simulink model "gm_sampleModel1948_1_sub"  (R2023a)
settings: Solver=VariableStepAuto  StartTime=0.0  StopTime=10.0  RelTol=1e-3
libraries: simulink x3
settings Model: Creator=user1  LastModifiedBy=user1
settings OptimizationCC: BlockReduction=off  ConditionallyExecuteInputs=off
settings DebuggingCC: InheritedTsInSrcMsg=none

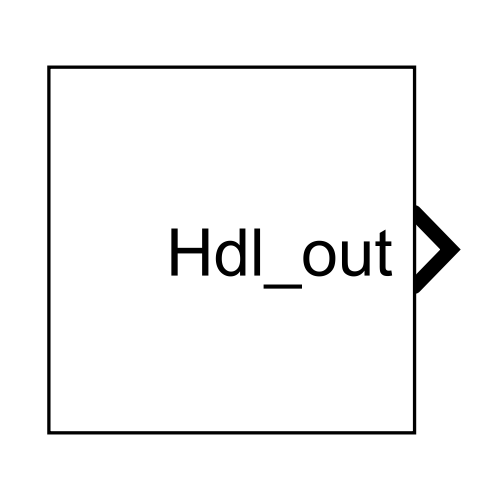
[thumbnail: Simulink's stored preview of the top-level diagram]
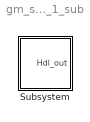
== system gm_sampleModel1948_1_sub ==
  Subsystem : Subsystem

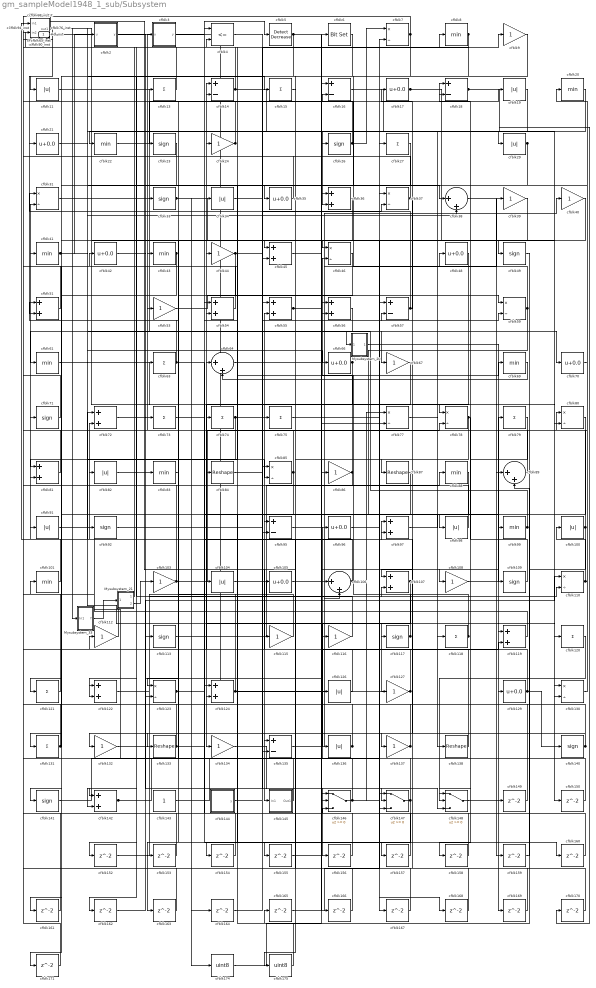
== system gm_sampleModel1948_1_sub/Subsystem ==
  Mysubsystem_20 : Subsystem
  Mysubsystem_21 : Subsystem
  Mysubsystem_33 : Subsystem
  cfblk{11,19,29,34,82,91,98,100,104,126,136} (11 alike) : Abs  OutDataTypeStr=uint8  SaturateOnIntegerOverflow=off
  cfblk{8,20,22,41,43,61,69,83,88,99,101} (11 alike) : MinMax  OutDataTypeStr=uint8
  cfblk102_inst : Subsystem
  cfblk{9,24,39..40,44,53,67,86,103,108,112,115..116,127,132,134,137} (17 alike) : Gain  OutDataTypeStr=uint8
  cfblk{17,21,35,42,48,66,70,96,105,129} (10 alike) : Bias  Bias=0.0  SaturateOnIntegerOverflow=off
  cfblk{38,64,89,106} (4 alike) : Sum  Inputs=|++  OutDataTypeStr=uint8
  cfblk{36,45,51,54..56,72,81,97,107,119,122,124,142} (14 alike) : Sum  OutDataTypeStr=uint8
  cfblk{23,26,33,49,71,92,109,113,117,140..141} (11 alike) : Signum
  cfblk10_inst : Subsystem
  cfblk{7,31,37,46,59,77..78,80,85,110,123,130} (12 alike) : Product  Inputs=*/  OutDataTypeStr=uint8  RndMeth=Zero  SaturateOnIntegerOverflow=on
  cfblk111_inst : Subsystem
  cfblk{13,15,27,63,73..75,79,118,120..121,131} (12 alike) : Sum  Inputs=+  OutDataTypeStr=uint8
  cfblk125_inst : Subsystem
  cfblk128_inst : Subsystem
  cfblk12_inst : Subsystem
  cfblk{84,87,133,138} (4 alike) : Reshape
  cfblk{14,16,18,57,95,135} (6 alike) : Sum  Inputs=+-  OutDataTypeStr=uint8
  cfblk139_inst : Subsystem
  cfblk143 : Constant  OutDataTypeStr=uint8  SampleTime=-1
  cfblk144 : Subsystem  mask(Counter Free-Running){NumBits=double(16), tsamp=double(-1)}
      mask prompts: NumBits "Simulink:masks:NumberOfBits_MP"; tsamp "Simulink:masks:SampleTime_MP"
      mask help: Simulink:masks:CounterFreeRunning_MD
  cfblk145 : Subsystem
  cfblk146 : Switch  OutDataTypeStr=uint8  SaturateOnIntegerOverflow=off  InputSameDT=off
  cfblk147 : Switch  OutDataTypeStr=uint8  SaturateOnIntegerOverflow=off  InputSameDT=off
  cfblk148 : Switch  OutDataTypeStr=uint8  SaturateOnIntegerOverflow=off  InputSameDT=off
  cfblk{149..150,152..171} (22 alike) : Delay  SampleTime=1
  cfblk174 : DataTypeConversion  OutDataTypeStr=uint8  SaturateOnIntegerOverflow=off  RndMeth=Floor
  cfblk175 : DataTypeConversion  OutDataTypeStr=uint8  SaturateOnIntegerOverflow=off  RndMeth=Floor
  cfblk2 : Subsystem  mask(Compare To Constant){relop=<=, const=double(3), OutDataTypeStr=uint8, ZeroCross=on}
      mask prompts: relop "Simulink:masks:Operator_MP"; const "Simulink:masks:ConstantValue_MP"; OutDataTypeStr "Simulink:masks:OutputDataType_MP"; ZeroCross "Simulink:masks:EnableZerocrossingDetection_MP"
      mask help: Simulink:masks:CompareToConstant_MD
      mask init:
      | OutDataTypeStr = 'uint8';
      | ZeroCross = 'on';
      | blkName = 'sampleModel1948_1_sub/Subsystem/cfblk2';
      | const = double(3);
      | const_str = '3.0';
      | const_val = double(3);
      | relop = '<=';
      | setValue = 'fixdt(0, 8)';
      | str = '<= 3';
      mask TypeOptions relop: == | ~= | < | <= | >= | >
      mask TypeOptions OutDataTypeStr: Simulink:masks:uint8 | Simulink:masks:boolean
      mask Callback ZeroCross: sl('zeroCrossEnable', gcbh);
      mask Display: disp(str)
  cfblk28_inst : Subsystem
  cfblk3 : Subsystem  mask(Compare To Constant){relop=<=, const=double(3), OutDataTypeStr=uint8, ZeroCross=on}
      mask prompts: relop "Simulink:masks:Operator_MP"; const "Simulink:masks:ConstantValue_MP"; OutDataTypeStr "Simulink:masks:OutputDataType_MP"; ZeroCross "Simulink:masks:EnableZerocrossingDetection_MP"
      mask help: Simulink:masks:CompareToConstant_MD
      mask init:
      | OutDataTypeStr = 'uint8';
      | ZeroCross = 'on';
      | blkName = 'sampleModel1948_1_sub/Subsystem/cfblk3';
      | const = double(3);
      | const_str = '3.0';
      | const_val = double(3);
      | relop = '<=';
      | setValue = 'fixdt(0, 8)';
      | str = '<= 3';
      mask TypeOptions relop: == | ~= | < | <= | >= | >
      mask TypeOptions OutDataTypeStr: Simulink:masks:uint8 | Simulink:masks:boolean
      mask Callback ZeroCross: sl('zeroCrossEnable', gcbh);
      mask Display: disp(str)
  cfblk30_inst : Subsystem
  cfblk32_inst : Subsystem
  cfblk4 : RelationalOperator  Operator=<=  OutDataTypeStr=boolean  InputSameDT=off
  cfblk47_inst : Subsystem
  cfblk5 : simulink/Logic and Bit Operations/Detect Decrease  vinit=0.0  OutDataTypeStr=uint8
      settings: LibrarySourceBlock=|
      | hdlsllib/Logic and Bit
      | Operations/Detect
      | Decrease
  cfblk58_inst : Subsystem
  cfblk6 : simulink/Logic and Bit Operations/Bit Set  iBit=0
      settings: LibrarySourceBlock=|
      | hdlsllib/Logic and Bit
      | Operations/Bit Set
  cfblk60_inst : Subsystem
  cfblk62_inst : Subsystem
  cfblk65_inst : Subsystem
  cfblk68_inst : Subsystem
  cfblk76_inst : Subsystem
  cfblk90_inst : Subsystem
  cfblk94_inst : Subsystem
  Hdl_out : Outport  OutDataTypeStr=uint8  SampleTime=1
  wires:
  Mysubsystem_20/1(Out1) -> cfblk169/1
  Mysubsystem_21/1(Out1) -> cfblk60_inst/2(in2)
  Mysubsystem_21/2(Out2) -> cfblk103/1
  Mysubsystem_33/1(Y) -> Mysubsystem_21/1(In1)
  cfblk10_inst/1(out1) -> cfblk11/1
  cfblk100/1 -> cfblk165/1, cfblk3/1(u)
  cfblk101/1 -> cfblk62_inst/1(in1)
  cfblk102_inst/1(out1) -> cfblk145/1(In1)
  cfblk103/1 -> cfblk94_inst/1(in1), cfblk78/2
  cfblk104/1 -> cfblk107/2
  cfblk105/1 -> cfblk40/1
  cfblk106/1 -> cfblk72/2, cfblk31/2
  cfblk107/1 -> cfblk155/1, cfblk134/1
  cfblk108/1 -> cfblk79/1
  cfblk109/1 -> cfblk48/1
  cfblk11/1 -> cfblk70/1
  cfblk110/1 -> cfblk35/1, cfblk100/1
  cfblk111_inst/1(out1) -> cfblk139_inst/1(in1), cfblk124/2
  cfblk112/1 -> cfblk47_inst/1(in1)
  cfblk113/1 -> cfblk88/1
  cfblk115/1 -> cfblk53/1
  cfblk116/1 -> cfblk58_inst/1(in1)
  cfblk117/1 -> cfblk42/1, cfblk31/1
  cfblk118/1 -> cfblk111_inst/1(in1), cfblk46/2
  cfblk119/1 -> cfblk101/1
  cfblk12_inst/1(out1) -> cfblk73/1
  cfblk120/1 -> cfblk148/2
  cfblk121/1 -> cfblk12_inst/1(in1)
  cfblk122/1 -> cfblk110/2
  cfblk123/1 -> cfblk174/1, cfblk157/1
  cfblk124/1 -> cfblk14/1, cfblk106/2
  cfblk125_inst/1(out1) -> cfblk49/1
  cfblk126/1 -> cfblk128_inst/1(in1)
  cfblk127/1 -> cfblk55/2, cfblk30_inst/1(in1), cfblk44/1, Hdl_out/1
  cfblk128_inst/1(out1) -> Mysubsystem_33/1(In1)
  cfblk129/1 -> cfblk54/2, cfblk140/1
  cfblk13/1 -> cfblk65_inst/1(in1)
  cfblk130/1 -> cfblk80/1
  cfblk131/1 -> cfblk128_inst/2(in2), cfblk41/1
  cfblk132/1 -> cfblk4/1
  cfblk133/1 -> cfblk97/1, cfblk71/1
  cfblk134/1 -> cfblk156/1
  cfblk135/1 -> cfblk39/1
  cfblk136/1 -> cfblk30_inst/2(in2), cfblk135/1
  cfblk137/1 -> cfblk94_inst/2(in2), cfblk91/1, cfblk24/1
  cfblk138/1 -> cfblk82/1
  cfblk139_inst/1(out1) -> cfblk86/1
  cfblk14/1 -> cfblk76_inst/2(in2), cfblk29/1
  cfblk140/1 -> cfblk132/1, cfblk43/1
  cfblk141/1 -> cfblk45/2
  cfblk142/1 -> cfblk96/1, cfblk57/1
  cfblk143/1 -> cfblk56/1
  cfblk144/1(y) -> cfblk59/2
  cfblk145/1(Out1) -> cfblk72/1
  cfblk146/1 -> cfblk12_inst/2(in2), cfblk77/1, cfblk7/2, cfblk27/1
  cfblk147/1 -> cfblk106/1, cfblk163/1, cfblk13/1
  cfblk148/1 -> cfblk149/1
  cfblk149/1 -> cfblk139_inst/2(in2)
  cfblk15/1 -> cfblk45/1
  cfblk150/1 -> cfblk111_inst/2(in2)
  cfblk152/1 -> cfblk64/1
  cfblk153/1 -> cfblk62_inst/2(in2)
  cfblk154/1 -> cfblk124/1
  cfblk155/1 -> cfblk119/2
  cfblk156/1 -> cfblk146/3
  cfblk157/1 -> cfblk14/2
  cfblk158/1 -> cfblk32_inst/2(in2)
  cfblk159/1 -> cfblk89/2
  cfblk16/1 -> cfblk120/1
  cfblk160/1 -> cfblk76_inst/1(in1)
  cfblk161/1 -> cfblk60_inst/1(in1)
  cfblk162/1 -> cfblk110/1
  cfblk163/1 -> cfblk90_inst/2(in2)
  cfblk164/1 -> cfblk57/2
  cfblk165/1 -> cfblk37/1
  cfblk166/1 -> cfblk125_inst/2(in2)
  cfblk167/1 -> cfblk95/1
  cfblk168/1 -> cfblk146/1
  cfblk169/1 -> cfblk4/2
  cfblk17/1 -> cfblk89/1, cfblk130/2
  cfblk170/1 -> cfblk97/2
  cfblk171/1 -> cfblk58_inst/2(in2)
  cfblk174/1 -> cfblk6/1
  cfblk175/1 -> cfblk104/1
  cfblk18/1 -> cfblk170/1, cfblk130/1
  cfblk19/1 -> cfblk122/2
  cfblk2/1(y) -> cfblk147/2
  cfblk20/1 -> cfblk22/1
  cfblk21/1 -> cfblk66/1
  cfblk22/1 -> cfblk19/1
  cfblk23/1 -> cfblk161/1
  cfblk24/1 -> cfblk68_inst/2(in2), cfblk10_inst/2(in2)
  cfblk26/1 -> cfblk125_inst/1(in1), cfblk7/1
  cfblk27/1 -> cfblk84/1
  cfblk28_inst/1(out1) -> cfblk92/1, cfblk36/2, cfblk123/2
  cfblk29/1 -> cfblk135/2, cfblk152/1
  cfblk3/1(y) -> cfblk5/1
  cfblk30_inst/1(out1) -> cfblk75/1
  cfblk31/1 -> cfblk56/2
  cfblk32_inst/1(out1) -> cfblk118/1
  cfblk33/1 -> cfblk147/1, cfblk164/1
  cfblk34/1 -> cfblk78/1
  cfblk35/1 -> cfblk23/1
  cfblk36/1 -> cfblk81/1
  cfblk37/1 -> cfblk90_inst/1(in1), cfblk87/1
  cfblk38/1 -> cfblk80/2
  cfblk39/1 -> cfblk153/1
  cfblk4/1 -> cfblk119/1
  cfblk40/1 -> cfblk46/1
  cfblk41/1 -> cfblk166/1, cfblk2/1(u)
  cfblk42/1 -> cfblk113/1
  cfblk43/1 -> cfblk142/1, cfblk171/1
  cfblk44/1 -> cfblk133/1, cfblk8/1
  cfblk45/1 -> cfblk108/1
  cfblk46/1 -> cfblk123/1
  cfblk47_inst/1(out1) -> cfblk102_inst/2(in2), cfblk150/1
  cfblk48/1 -> cfblk137/1
  cfblk49/1 -> cfblk129/1
  cfblk5/1 -> cfblk77/2, cfblk162/1
  cfblk51/1 -> cfblk10_inst/1(in1)
  cfblk53/1 -> cfblk59/1
  cfblk54/1 -> cfblk68_inst/1(in1)
  cfblk55/1 -> cfblk109/1, cfblk9/1
  cfblk56/1 -> cfblk61/1
  cfblk57/1 -> cfblk34/1, cfblk17/1
  cfblk58_inst/1(out1) -> cfblk26/1
  cfblk59/1 -> cfblk95/2, cfblk16/2
  cfblk6/1 -> cfblk175/1
  cfblk60_inst/1(out1) -> cfblk51/2, cfblk147/3, cfblk136/1, cfblk115/1
  cfblk61/1 -> cfblk159/1
  cfblk62_inst/1(out1) -> cfblk38/2, cfblk127/1
  cfblk63/1 -> cfblk98/1, cfblk51/1
  cfblk64/1 -> cfblk116/1
  cfblk65_inst/1(out1) -> cfblk15/1
  cfblk66/1 -> cfblk54/1, cfblk74/1
  cfblk67/1 -> cfblk146/2
  cfblk68_inst/1(out1) -> cfblk85/2, cfblk167/1
  cfblk69/1 -> cfblk64/2
  cfblk7/1 -> cfblk36/1, cfblk28_inst/1(in1), cfblk142/2
  cfblk70/1 -> cfblk20/1
  cfblk71/1 -> cfblk32_inst/1(in1)
  cfblk72/1 -> cfblk126/1
  cfblk73/1 -> cfblk160/1
  cfblk74/1 -> cfblk37/2, cfblk121/1
  cfblk75/1 -> cfblk18/1
  cfblk76_inst/1(out1) -> cfblk38/1, cfblk67/1
  cfblk77/1 -> cfblk138/1
  cfblk78/1 -> cfblk105/1, cfblk158/1
  cfblk79/1 -> cfblk148/1
  cfblk8/1 -> cfblk28_inst/2(in2), cfblk141/1
  cfblk80/1 -> cfblk122/1
  cfblk81/1 -> cfblk47_inst/2(in2)
  cfblk82/1 -> cfblk83/1
  cfblk83/1 -> cfblk33/1
  cfblk84/1 -> cfblk148/3
  cfblk85/1 -> cfblk102_inst/1(in1), cfblk154/1
  cfblk86/1 -> cfblk81/2, cfblk65_inst/2(in2)
  cfblk87/1 -> cfblk131/1
  cfblk88/1 -> cfblk107/1
  cfblk89/1 -> cfblk55/1
  cfblk9/1 -> cfblk112/1
  cfblk90_inst/1(out1) -> cfblk63/1
  cfblk91/1 -> cfblk117/1
  cfblk92/1 -> cfblk85/1
  cfblk94_inst/1(out1) -> cfblk21/1
  cfblk95/1 -> cfblk69/1
  cfblk96/1 -> cfblk168/1
  cfblk97/1 -> cfblk99/1
  cfblk98/1 -> cfblk16/1
  cfblk99/1 -> cfblk18/2, Mysubsystem_20/1(In1)

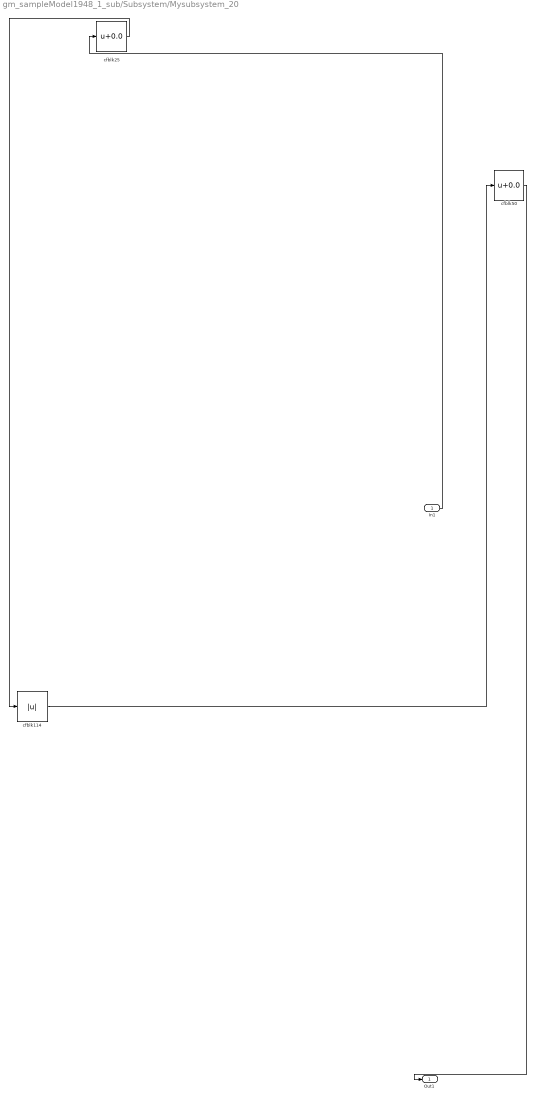
== system gm_sampleModel1948_1_sub/Subsystem/Mysubsystem_20 ==
  In1 : Inport  OutDataTypeStr=uint8  PortDimensions=1  SampleTime=1
  cfblk114 : Abs  SaturateOnIntegerOverflow=off
  cfblk25 : Bias  Bias=0.0  SaturateOnIntegerOverflow=off
  cfblk50 : Bias  Bias=0.0  SaturateOnIntegerOverflow=off
  Out1 : Outport  SampleTime=1
  wires:
  In1/1 -> cfblk25/1
  cfblk114/1 -> cfblk50/1
  cfblk25/1 -> cfblk114/1
  cfblk50/1 -> Out1/1

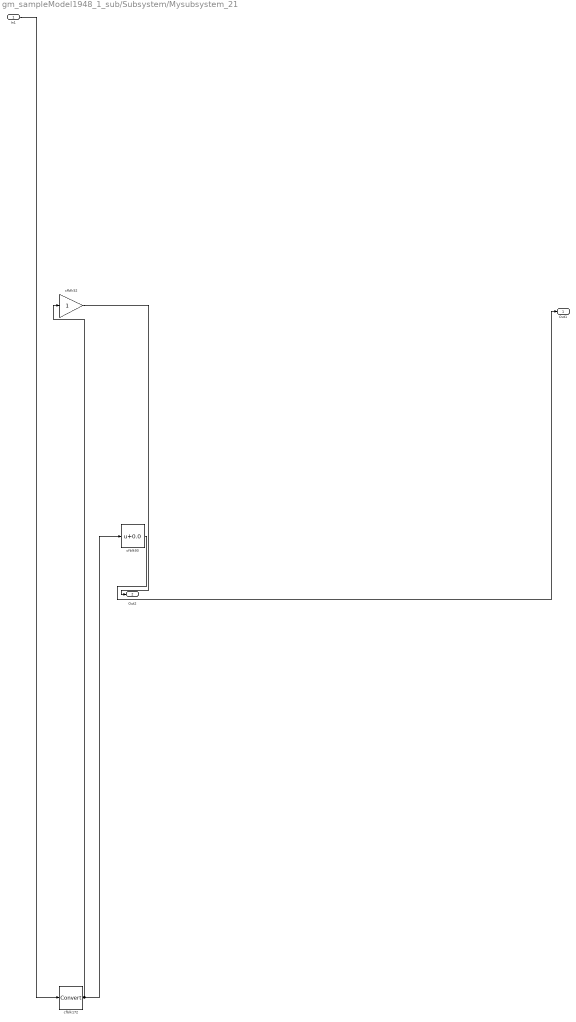
== system gm_sampleModel1948_1_sub/Subsystem/Mysubsystem_21 ==
  In1 : Inport  OutDataTypeStr=boolean  PortDimensions=1  SampleTime=1
  cfblk172 : DataTypeConversion  SaturateOnIntegerOverflow=off  RndMeth=Floor
  cfblk52 : Gain
  cfblk93 : Bias  Bias=0.0  SaturateOnIntegerOverflow=off
  Out1 : Outport  SampleTime=1
  Out2 : Outport  Port=2  SampleTime=1
  wires:
  In1/1 -> cfblk172/1
  cfblk172/1 -> cfblk93/1, cfblk52/1
  cfblk52/1 -> Out2/1
  cfblk93/1 -> Out1/1

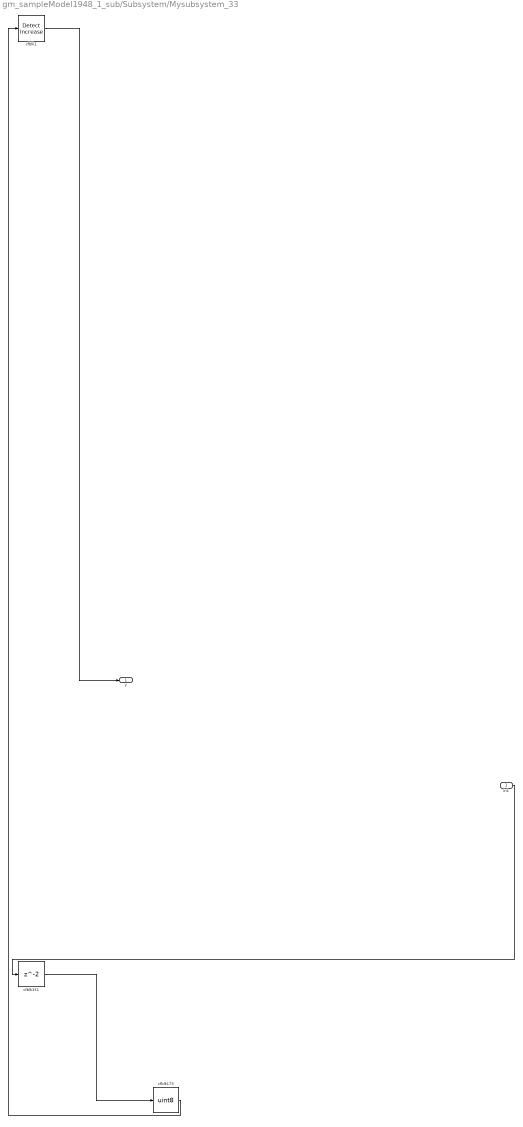
== system gm_sampleModel1948_1_sub/Subsystem/Mysubsystem_33 ==
  In1 : Inport  OutDataTypeStr=uint8  PortDimensions=1  SampleTime=1
  cfblk1 : simulink/Logic and Bit Operations/Detect Increase  vinit=0.0  OutDataTypeStr=boolean
      settings: LibrarySourceBlock=|
      | hdlsllib/Logic and Bit
      | Operations/Detect
      | Increase
  cfblk151 : Delay  SampleTime=1
  cfblk173 : DataTypeConversion  OutDataTypeStr=uint8  SaturateOnIntegerOverflow=off  RndMeth=Floor
  Y : Outport  SampleTime=1
  wires:
  In1/1 -> cfblk151/1
  cfblk1/1 -> Y/1
  cfblk151/1 -> cfblk173/1
  cfblk173/1 -> cfblk1/1

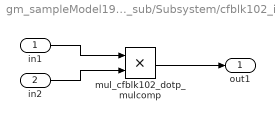
== system gm_sampleModel1948_1_sub/Subsystem/cfblk102_inst ==
  in1 : Inport  OutDataTypeStr=uint8  SampleTime=1
  in2 : Inport  Port=2  OutDataTypeStr=uint8  SampleTime=1
  mul_cfblk102_dotp_mulcomp : Product  Inputs=**  OutDataTypeStr=uint8  SampleTime=1
  out1 : Outport  OutDataTypeStr=uint8  SampleTime=1
  wires:
  in1/1 -> mul_cfblk102_dotp_mulcomp/1
  in2/1 -> mul_cfblk102_dotp_mulcomp/2
  mul_cfblk102_dotp_mulcomp/1 -> out1/1

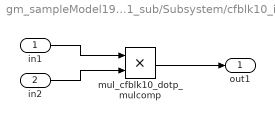
== system gm_sampleModel1948_1_sub/Subsystem/cfblk10_inst ==
  in1 : Inport  OutDataTypeStr=uint8  SampleTime=1
  in2 : Inport  Port=2  OutDataTypeStr=uint8  SampleTime=1
  mul_cfblk10_dotp_mulcomp : Product  Inputs=**  OutDataTypeStr=uint8  SampleTime=1
  out1 : Outport  OutDataTypeStr=uint8  SampleTime=1
  wires:
  in1/1 -> mul_cfblk10_dotp_mulcomp/1
  in2/1 -> mul_cfblk10_dotp_mulcomp/2
  mul_cfblk10_dotp_mulcomp/1 -> out1/1

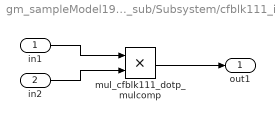
== system gm_sampleModel1948_1_sub/Subsystem/cfblk111_inst ==
  in1 : Inport  OutDataTypeStr=uint8  SampleTime=1
  in2 : Inport  Port=2  OutDataTypeStr=uint8  SampleTime=1
  mul_cfblk111_dotp_mulcomp : Product  Inputs=**  OutDataTypeStr=uint8  SampleTime=1
  out1 : Outport  OutDataTypeStr=uint8  SampleTime=1
  wires:
  in1/1 -> mul_cfblk111_dotp_mulcomp/1
  in2/1 -> mul_cfblk111_dotp_mulcomp/2
  mul_cfblk111_dotp_mulcomp/1 -> out1/1

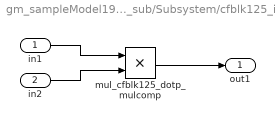
== system gm_sampleModel1948_1_sub/Subsystem/cfblk125_inst ==
  in1 : Inport  OutDataTypeStr=uint8  SampleTime=1
  in2 : Inport  Port=2  OutDataTypeStr=uint8  SampleTime=1
  mul_cfblk125_dotp_mulcomp : Product  Inputs=**  OutDataTypeStr=uint8  SampleTime=1
  out1 : Outport  OutDataTypeStr=uint8  SampleTime=1
  wires:
  in1/1 -> mul_cfblk125_dotp_mulcomp/1
  in2/1 -> mul_cfblk125_dotp_mulcomp/2
  mul_cfblk125_dotp_mulcomp/1 -> out1/1

== system gm_sampleModel1948_1_sub/Subsystem/cfblk128_inst ==
  in1 : Inport  OutDataTypeStr=uint8  SampleTime=1
  in2 : Inport  Port=2  OutDataTypeStr=uint8  SampleTime=1
  mul_cfblk128_dotp_mulcomp : Product  Inputs=**  OutDataTypeStr=uint8  SampleTime=1
  out1 : Outport  OutDataTypeStr=uint8  SampleTime=1
  wires:
  in1/1 -> mul_cfblk128_dotp_mulcomp/1
  in2/1 -> mul_cfblk128_dotp_mulcomp/2
  mul_cfblk128_dotp_mulcomp/1 -> out1/1

== system gm_sampleModel1948_1_sub/Subsystem/cfblk12_inst ==
  in1 : Inport  OutDataTypeStr=uint8  SampleTime=1
  in2 : Inport  Port=2  OutDataTypeStr=uint8  SampleTime=1
  mul_cfblk12_dotp_mulcomp : Product  Inputs=**  OutDataTypeStr=uint8  SampleTime=1
  out1 : Outport  OutDataTypeStr=uint8  SampleTime=1
  wires:
  in1/1 -> mul_cfblk12_dotp_mulcomp/1
  in2/1 -> mul_cfblk12_dotp_mulcomp/2
  mul_cfblk12_dotp_mulcomp/1 -> out1/1

== system gm_sampleModel1948_1_sub/Subsystem/cfblk139_inst ==
  in1 : Inport  OutDataTypeStr=uint8  SampleTime=1
  in2 : Inport  Port=2  OutDataTypeStr=uint8  SampleTime=1
  mul_cfblk139_dotp_mulcomp : Product  Inputs=**  OutDataTypeStr=uint8  SampleTime=1
  out1 : Outport  OutDataTypeStr=uint8  SampleTime=1
  wires:
  in1/1 -> mul_cfblk139_dotp_mulcomp/1
  in2/1 -> mul_cfblk139_dotp_mulcomp/2
  mul_cfblk139_dotp_mulcomp/1 -> out1/1

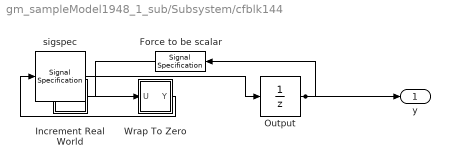
== system gm_sampleModel1948_1_sub/Subsystem/cfblk144 ==
  Force to be scalar : SignalSpecification  DisableCoverage=on  Dimensions=1
  Increment Real World : Subsystem  mask(Real World Value Increment){}
      mask help: Simulink:masks:RealWorldValueIncrement_MD
      mask Display: disp('V++')
  Output : UnitDelay  InitialCondition=0.0  SampleTime=tsamp  HasFrameUpgradeWarning=on
  Wrap To Zero : Subsystem  mask(Wrap To Zero){Threshold=double(65535)}
      mask prompts: Threshold "Simulink:masks:Threshold_MP"
      mask help: Simulink:masks:WrapToZero_MD
  sigspec : SignalSpecification  OutDataTypeStr=uint16  Dimensions=1
  y : Outport  SampleTime=1
  wires:
  Force to be scalar/1 -> Increment Real World/1(u)
  Increment Real World/1(y) -> Wrap To Zero/1(U)
  Output/1 -> Force to be scalar/1, y/1
  Wrap To Zero/1(Y) -> sigspec/1
  sigspec/1 -> Output/1

== system gm_sampleModel1948_1_sub/Subsystem/cfblk145 ==
  In1 : Inport  OutDataTypeStr=uint8  PortDimensions=1  SampleTime=1
  Out1 : Outport  SampleTime=1
  wires:
  In1/1 -> Out1/1

== system gm_sampleModel1948_1_sub/Subsystem/cfblk2 ==
  u : Inport  OutDataTypeStr=uint8  SampleTime=1
  Compare : RelationalOperator  Operator=<=  OutDataTypeStr=fixdt(0, 8)
  Constant : Constant  DisableCoverage=on  Value=const  OutDataTypeStr=Inherit: Inherit via back propagation  SampleTime=-1
  y : Outport  SampleTime=1
  wires:
  u/1 -> Compare/1
  Compare/1 -> y/1
  Constant/1 -> Compare/2

== system gm_sampleModel1948_1_sub/Subsystem/cfblk28_inst ==
  in1 : Inport  OutDataTypeStr=uint8  SampleTime=1
  in2 : Inport  Port=2  OutDataTypeStr=uint8  SampleTime=1
  mul_cfblk28_dotp_mulcomp : Product  Inputs=**  OutDataTypeStr=uint8  SampleTime=1
  out1 : Outport  OutDataTypeStr=uint8  SampleTime=1
  wires:
  in1/1 -> mul_cfblk28_dotp_mulcomp/1
  in2/1 -> mul_cfblk28_dotp_mulcomp/2
  mul_cfblk28_dotp_mulcomp/1 -> out1/1

== system gm_sampleModel1948_1_sub/Subsystem/cfblk3 ==
  u : Inport  OutDataTypeStr=uint8  SampleTime=1
  Compare : RelationalOperator  Operator=<=  OutDataTypeStr=fixdt(0, 8)
  Constant : Constant  DisableCoverage=on  Value=const  OutDataTypeStr=Inherit: Inherit via back propagation  SampleTime=-1
  y : Outport  SampleTime=1
  wires:
  u/1 -> Compare/1
  Compare/1 -> y/1
  Constant/1 -> Compare/2

== system gm_sampleModel1948_1_sub/Subsystem/cfblk30_inst ==
  in1 : Inport  OutDataTypeStr=uint8  SampleTime=1
  in2 : Inport  Port=2  OutDataTypeStr=uint8  SampleTime=1
  mul_cfblk30_dotp_mulcomp : Product  Inputs=**  OutDataTypeStr=uint8  SampleTime=1
  out1 : Outport  OutDataTypeStr=uint8  SampleTime=1
  wires:
  in1/1 -> mul_cfblk30_dotp_mulcomp/1
  in2/1 -> mul_cfblk30_dotp_mulcomp/2
  mul_cfblk30_dotp_mulcomp/1 -> out1/1

== system gm_sampleModel1948_1_sub/Subsystem/cfblk32_inst ==
  in1 : Inport  OutDataTypeStr=uint8  SampleTime=1
  in2 : Inport  Port=2  OutDataTypeStr=uint8  SampleTime=1
  mul_cfblk32_dotp_mulcomp : Product  Inputs=**  OutDataTypeStr=uint8  SampleTime=1
  out1 : Outport  OutDataTypeStr=uint8  SampleTime=1
  wires:
  in1/1 -> mul_cfblk32_dotp_mulcomp/1
  in2/1 -> mul_cfblk32_dotp_mulcomp/2
  mul_cfblk32_dotp_mulcomp/1 -> out1/1

== system gm_sampleModel1948_1_sub/Subsystem/cfblk47_inst ==
  in1 : Inport  OutDataTypeStr=uint8  SampleTime=1
  in2 : Inport  Port=2  OutDataTypeStr=uint8  SampleTime=1
  mul_cfblk47_dotp_mulcomp : Product  Inputs=**  OutDataTypeStr=uint8  SampleTime=1
  out1 : Outport  OutDataTypeStr=uint8  SampleTime=1
  wires:
  in1/1 -> mul_cfblk47_dotp_mulcomp/1
  in2/1 -> mul_cfblk47_dotp_mulcomp/2
  mul_cfblk47_dotp_mulcomp/1 -> out1/1

== system gm_sampleModel1948_1_sub/Subsystem/cfblk58_inst ==
  in1 : Inport  OutDataTypeStr=uint8  SampleTime=1
  in2 : Inport  Port=2  OutDataTypeStr=uint8  SampleTime=1
  mul_cfblk58_dotp_mulcomp : Product  Inputs=**  OutDataTypeStr=uint8  SampleTime=1
  out1 : Outport  OutDataTypeStr=uint8  SampleTime=1
  wires:
  in1/1 -> mul_cfblk58_dotp_mulcomp/1
  in2/1 -> mul_cfblk58_dotp_mulcomp/2
  mul_cfblk58_dotp_mulcomp/1 -> out1/1

== system gm_sampleModel1948_1_sub/Subsystem/cfblk60_inst ==
  in1 : Inport  OutDataTypeStr=uint8  SampleTime=1
  in2 : Inport  Port=2  OutDataTypeStr=uint8  SampleTime=1
  mul_cfblk60_dotp_mulcomp : Product  Inputs=**  OutDataTypeStr=uint8  SampleTime=1
  out1 : Outport  OutDataTypeStr=uint8  SampleTime=1
  wires:
  in1/1 -> mul_cfblk60_dotp_mulcomp/1
  in2/1 -> mul_cfblk60_dotp_mulcomp/2
  mul_cfblk60_dotp_mulcomp/1 -> out1/1

== system gm_sampleModel1948_1_sub/Subsystem/cfblk62_inst ==
  in1 : Inport  OutDataTypeStr=uint8  SampleTime=1
  in2 : Inport  Port=2  OutDataTypeStr=uint8  SampleTime=1
  mul_cfblk62_dotp_mulcomp : Product  Inputs=**  OutDataTypeStr=uint8  SampleTime=1
  out1 : Outport  OutDataTypeStr=uint8  SampleTime=1
  wires:
  in1/1 -> mul_cfblk62_dotp_mulcomp/1
  in2/1 -> mul_cfblk62_dotp_mulcomp/2
  mul_cfblk62_dotp_mulcomp/1 -> out1/1

== system gm_sampleModel1948_1_sub/Subsystem/cfblk65_inst ==
  in1 : Inport  OutDataTypeStr=uint8  SampleTime=1
  in2 : Inport  Port=2  OutDataTypeStr=uint8  SampleTime=1
  mul_cfblk65_dotp_mulcomp : Product  Inputs=**  OutDataTypeStr=uint8  SampleTime=1
  out1 : Outport  OutDataTypeStr=uint8  SampleTime=1
  wires:
  in1/1 -> mul_cfblk65_dotp_mulcomp/1
  in2/1 -> mul_cfblk65_dotp_mulcomp/2
  mul_cfblk65_dotp_mulcomp/1 -> out1/1

== system gm_sampleModel1948_1_sub/Subsystem/cfblk68_inst ==
  in1 : Inport  OutDataTypeStr=uint8  SampleTime=1
  in2 : Inport  Port=2  OutDataTypeStr=uint8  SampleTime=1
  mul_cfblk68_dotp_mulcomp : Product  Inputs=**  OutDataTypeStr=uint8  SampleTime=1
  out1 : Outport  OutDataTypeStr=uint8  SampleTime=1
  wires:
  in1/1 -> mul_cfblk68_dotp_mulcomp/1
  in2/1 -> mul_cfblk68_dotp_mulcomp/2
  mul_cfblk68_dotp_mulcomp/1 -> out1/1

== system gm_sampleModel1948_1_sub/Subsystem/cfblk76_inst ==
  in1 : Inport  OutDataTypeStr=uint8  SampleTime=1
  in2 : Inport  Port=2  OutDataTypeStr=uint8  SampleTime=1
  mul_cfblk76_dotp_mulcomp : Product  Inputs=**  OutDataTypeStr=uint8  SampleTime=1
  out1 : Outport  OutDataTypeStr=uint8  SampleTime=1
  wires:
  in1/1 -> mul_cfblk76_dotp_mulcomp/1
  in2/1 -> mul_cfblk76_dotp_mulcomp/2
  mul_cfblk76_dotp_mulcomp/1 -> out1/1

== system gm_sampleModel1948_1_sub/Subsystem/cfblk90_inst ==
  in1 : Inport  OutDataTypeStr=uint8  SampleTime=1
  in2 : Inport  Port=2  OutDataTypeStr=uint8  SampleTime=1
  mul_cfblk90_dotp_mulcomp : Product  Inputs=**  OutDataTypeStr=uint8  SampleTime=1
  out1 : Outport  OutDataTypeStr=uint8  SampleTime=1
  wires:
  in1/1 -> mul_cfblk90_dotp_mulcomp/1
  in2/1 -> mul_cfblk90_dotp_mulcomp/2
  mul_cfblk90_dotp_mulcomp/1 -> out1/1

== system gm_sampleModel1948_1_sub/Subsystem/cfblk94_inst ==
  in1 : Inport  OutDataTypeStr=uint8  SampleTime=1
  in2 : Inport  Port=2  OutDataTypeStr=uint8  SampleTime=1
  mul_cfblk94_dotp_mulcomp : Product  Inputs=**  OutDataTypeStr=uint8  SampleTime=1
  out1 : Outport  OutDataTypeStr=uint8  SampleTime=1
  wires:
  in1/1 -> mul_cfblk94_dotp_mulcomp/1
  in2/1 -> mul_cfblk94_dotp_mulcomp/2
  mul_cfblk94_dotp_mulcomp/1 -> out1/1

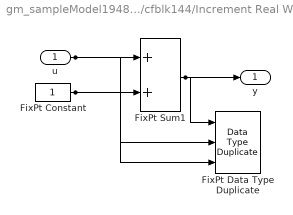
== system gm_sampleModel1948_1_sub/Subsystem/cfblk144/Increment Real World ==
  u : Inport  OutDataTypeStr=uint16  SampleTime=1
  FixPt Constant : Constant  DisableCoverage=on  OutDataTypeStr=Inherit: Inherit via back propagation  SampleTime=-1
  FixPt Data Type Duplicate : DataTypeDuplicate  DisableCoverage=on  NumInputPorts=3
  FixPt Sum1 : Sum  InputSameDT=on  OutDataTypeStr=Inherit: Inherit via back propagation  LockScale=on
  y : Outport  SampleTime=1
  wires:
  u/1 -> FixPt Sum1/1, FixPt Data Type Duplicate/2
  FixPt Constant/1 -> FixPt Sum1/2, FixPt Data Type Duplicate/3
  FixPt Sum1/1 -> FixPt Data Type Duplicate/1, y/1

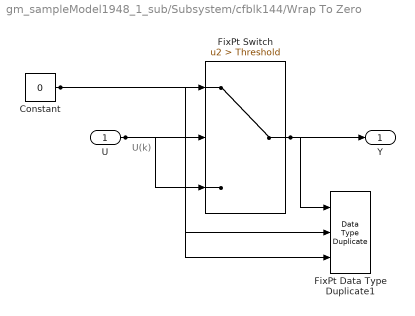
== system gm_sampleModel1948_1_sub/Subsystem/cfblk144/Wrap To Zero ==
  note: U(k)
  U : Inport  OutDataTypeStr=uint16  SampleTime=1
  Constant : Constant  DisableCoverage=on  Value=0  OutDataTypeStr=Inherit: Inherit via back propagation  SampleTime=-1
  FixPt Data Type Duplicate1 : DataTypeDuplicate  DisableCoverage=on  NumInputPorts=3
  FixPt Switch : Switch  Criteria=u2 > Threshold  Threshold=Threshold  OutDataTypeStr=Inherit: Inherit via back propagation  ZeroCross=off  SaturateOnIntegerOverflow=off  InputSameDT=off
  Y : Outport  SampleTime=1
  wires:
  U/1 -> FixPt Switch/3, FixPt Switch/2, FixPt Data Type Duplicate1/2
  Constant/1 -> FixPt Switch/1, FixPt Data Type Duplicate1/3
  FixPt Switch/1 -> FixPt Data Type Duplicate1/1, Y/1
